simulink model "Select_PI_for_FOC_of_IM"  (R2017b)
settings: Solver=FixedStepDiscrete  StartTime=0.0  StopTime=10.0  FixedStep=Ts  MaxStep=1e-4  RelTol=1e-3
InitFcn:
  | Ts = 2e-5; Fsw = 2e3;
  | %Motor 1
  | %===========================
  | %Pn = 15e3; Nn = 1460; Tn = 9.55*Pn/Nn;
  | %Rs = 0.2147; Lls = 0.000991;
  | %Rr = 0.2205; Llr = 0.000991;
  | %Lm = 0.06419;
  | %Ls = Lls + Lm;
  | %Lr = Llr + Lm;
  | %P = 4;
  | %J = 0.102;  B = 0.009541;
  | %===========================
  | % Motor 2
  | %===========================
  | Pn = 7.5e3; Nn = 1440; Tn = 9.55*Pn/Nn;
  | Rs = 0.7384; Lls = 0.003045;
  | Rr = 0.7402; Llr = 0.003045;
  | Lm = 0.1241;
  | Ls = Lls + Lm;
  | Lr = Llr + Lm;
  | P = 4;  %poles
  | J = 0.0343;  B = 0.000503;
  | %===========================
  | Tor = (Llr+Lm) /Rr;
  | sigma = 1 - Lm*Lm/(Ls*Lr);
  | Kpdq = (Rs+Rr*(Lm/Lr)^2)*2*pi*50;
  | Kidq  = sigma*Ls*2*pi*50;
  | Ids_ref = 220*sqrt(2)/sqrt(Rs^2+(2*pi*50*Ls)^2);
  | KT = (3/2)*(P/2)*(Lm^2/Lr)*Ids_ref;
  | %Kpw = J*2*pi*50/KT;
  | %Kiw = Kpw*2*pi*50/5;
  | Zt = 0.8; W_n = 2*pi*5;
  | Kpw = (2*Zt*W_n*J-B);
  | Kiw  = (J*W_n^2);
  | Nze = 1e-3;
undefined symbols (not defined in the file): DiscIntNeverNeededParam, Vdc
libraries: powerlib x4, powerlib_meascontrol x3, peGeneralControl x1
settings Model: Creator=ADMIN  LastModifiedBy=ADMIN

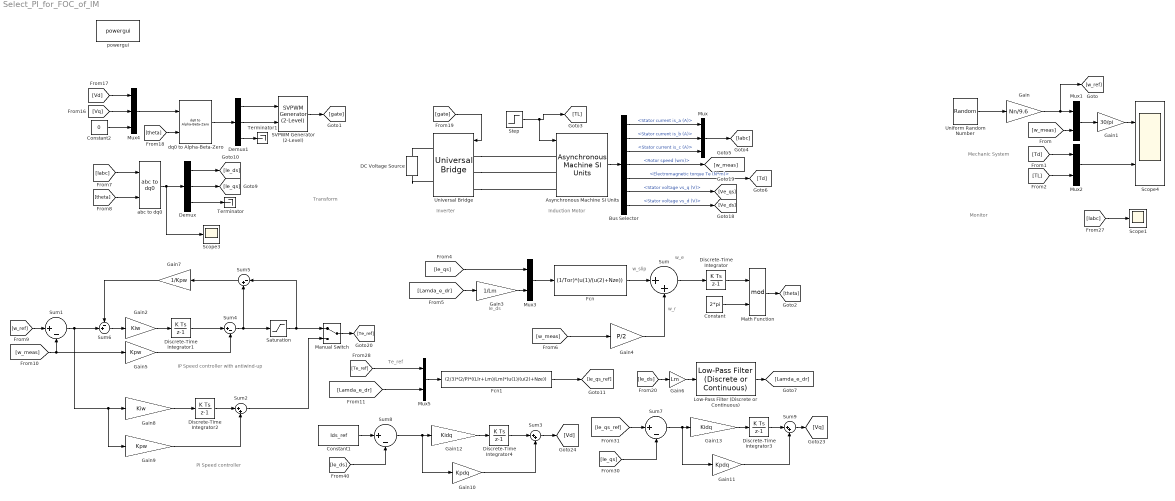
== system Select_PI_for_FOC_of_IM ==
  note: Monitor
  note: Induction Motor
  note: Transform
  note: Inverter
  note: Mechanic System
  note: Te_ref
  note: Ie_ds
  note: w_r
  note: w_slip
  note: w_e
  note: PI Speed controller
  note: IP Speed controller with antiwind-up
  Asynchronous Machine SI Units : powerlib/Machines/Asynchronous Machine SI Units  RotorType=Squirrel-cage  PresetModel="16:  10 HP (7.5KW)  400 V 50Hz 1440 RPM"  MechanicalLoad=Torque Tm  ShowDetailedParameters=on  ReferenceFrame=Synchronous  Units=SI  MeasurementBus=off  NominalParameters=[7500 400 50]  Stator=[0.7384 0.003045]  Rotor=[0.7402 0.003045]  Cage1=[0.4155 0.002066]  Cage2=[0.4168 0.0003495]  Lm=0.1241  Mechanical=[0.0343 0.000503 2]  PolePairs=2  InitialConditions=[1 0 0 0 0 0 0 0]  SimulateSaturation=off  Saturation=[14.03593122, 27.81365428, 53.79336849, 72.68890987, 97.98006896, 148.6815601, 215.7428561, 302.9841135, 428.7778367 ; 230, 322, 414, 460, 506, 552, 598, 644, 690]  LoadFlowParameters=1492000  TsPowergui=0  TsBlock=-1  IterativeModel=Trapezoidal non iterative  IterativeDiscreteModel=Trapezoidal non iterative  Pmec=0
  Bus Selector : BusSelector  OutputSignals=Stator measurements.Stator current is_a (A),Stator measurements.Stator current is_b (A),Stator measurements.Stator current is_c (A),Mechanical.Rotor speed (wm),Mechanical.Electromagnetic torque Te (N*m),Stator measurements.Stator voltage vs_q (V),Stator measurements.Stator voltage vs_d (V)
  Constant : Constant  Value=2*pi
  Constant1 : Constant  Value=Ids_ref
  Constant2 : Constant  Value=0
  DC Voltage Source : powerlib/Electrical Sources/DC Voltage Source  Amplitude=Vdc  Measurements=None
  Demux : Demux  Outputs=3
  Demux1 : Demux  Outputs=3
  Discrete-Time Integrator{,1..4} (5 alike) : DiscreteIntegrator  InitialConditionSetting=State (most efficient)  SampleTime=-1  ICPrevOutput=DiscIntNeverNeededParam  ICPrevScaledInput=DiscIntNeverNeededParam
  Fcn : Fcn  Expr=(1/Tor)*(u(1)/(u(2)+Nze))
  Fcn1 : Fcn  Expr=(2/3)*(2/P)*((Llr+Lm)/Lm)*(u(1)/(u(2)+Nze))
  Gain : Gain  Gain=Nn/9.6
  Gain1 : Gain  Gain=30/pi
  Gain10 : Gain  Gain=Kpdq
  Gain11 : Gain  Gain=Kpdq
  Gain12 : Gain  Gain=Kidq
  Gain13 : Gain  Gain=Kidq
  Gain2 : Gain  Gain=Kiw
  Gain3 : Gain  Gain=1/Lm
  Gain4 : Gain  Gain=P/2
  Gain5 : Gain  Gain=Kpw
  Gain6 : Gain  Gain=Lm
  Gain7 : Gain  Gain=1/Kpw
  Gain8 : Gain  Gain=Kiw
  Gain9 : Gain  Gain=Kpw
  Low-Pass Filter (Discrete or Continuous) : peGeneralControl/Low-Pass Filter (Discrete or Continuous)  K=1  T=Tor  B=inf  A=-inf  Ts=Ts
  Manual Switch : ManualSwitch
  Math Function : Math  Operator=mod  SaturateOnIntegerOverflow=on
  Mux : Mux  Inputs=3
  Mux{1..3,5} (4 alike) : Mux  Inputs=2
  Mux4 : Mux  Inputs=3
  SVPWM Generator (2-Level) : powerlib_meascontrol/Pulse & Signal Generators/SVPWM Generator (2-Level)  InputType=alpha-beta components  SwitchingPattern=Pattern #1  Fc=Fsw  ParUref=[0.8 -30 50]  Ts=Ts
      settings: SourceProductName=Simscape Power Systems  SourceProductBaseCode=PS
  Saturation : Saturate  UpperLimit=1.5*Tn  LowerLimit=-1.5*Tn
  Scope1 : Scope
  Scope3 : Scope
  Scope4 : Scope  NumInputPorts=2
  Step : Step  Time=5  Before=0.5*Tn  After=Tn  SampleTime=Ts
  Sum{,2..3,9} (4 alike) : Sum  Inputs=|++
  Sum{1,4,7..8} (4 alike) : Sum  Inputs=|+-
  Sum5 : Sum  Inputs=|-+
  Sum6 : Sum  Inputs=-+|
  Terminator : Terminator
  Terminator1 : Terminator
  Uniform Random Number : UniformRandomNumber  Minimum=0  Seed=5  SampleTime=2
  Universal Bridge : powerlib/Power Electronics/Universal Bridge  Arms=3  SnubberResistance=1e5  SnubberCapacitance=inf  Device=IGBT / Diodes  Ron=1e-3  Lon=0  ForwardVoltages="[  0  0  ]"  ForwardVoltage=0  GTOparameters=[ 10e-6 , 20e-6 ]  IGBTparameters=[ 1e-6 , 2e-6 ]  Measurements=None  Measurements_2=None  converterType=Rectifier
  abc to dq0 : powerlib_meascontrol/Transformations/abc to dq0  Alignment=90 degrees behind phase A axis
  dq0 to Alpha-Beta-Zero : powerlib_meascontrol/Transformations/dq0 to Alpha-Beta-Zero  Alignment=90 degrees behind phase A axis
      settings: SourceProductName=Simscape Power Systems  SourceProductBaseCode=PS
  powergui : powerlib/powergui  Priority=1  SimulationMode=Discrete  SampleTime=Ts  frequency=60  Iterations=50  frequencyindice=50  Pbase=100e6  ErrMax=1e-4  UnitsV=kV  UnitsW=MW  buscounter=0  FunctionMessages=off  echomessages=off  EnableUseOfTLC=off  CurrentSourceSwitches=off  DisableSnubberDevices=off  DisableRonSwitches=off  DisableVfSwitches=off  DisplayEquations=off  SolverType=Tustin/Backward Euler (TBE)  Interpol=off  ExternalGateDelay=off  methode=off  Ts=100  x0status=blocks  SPID=on  SwTol=0  HookPort=off  RestoreLinks=warning  ResistiveCurrentMeasurement=off  Frange=[0:2:500]  Ylog=off  Xlog=on  ShowGrid=off  save=off  variable=ZData  structure=IABC  ZoomFFT=off  StartTime=1.5  cycles=1  DisplayStyle=1  fundamental=6.7  FreqAxis=off  MaxFrequency=7000  frequencyindicesteady=1  RmsSteady=1  display=off
  wires:
  Step/1 -> [TL], Asynchronous Machine SI Units/1
  Demux/3 -> Terminator/1
  [TL] -> Mux2/2
  Fcn1/1 -> [Ie_qs_ref]
  Mux/1 -> [Iabc]
  Mux4/1 -> dq0 to Alpha-Beta-Zero/1
  dq0 to Alpha-Beta-Zero/1 -> Demux1/1
  Gain1/1 -> Scope4/1
  Demux1/1 -> SVPWM Generator (2-Level)/1
  [theta] -> abc to dq0/2
  Bus Selector/6 -> [Ve_qs]  "<Stator voltage vs_q (V)>"
  Saturation/1 -> Sum5/1, Manual Switch/1
  [gate] -> Universal Bridge/1
  Bus Selector/7 -> [Ve_ds]  "<Stator voltage vs_d (V)>"
  Demux/1 -> [Ie_ds]
  [w_meas] -> Gain4/1
  Demux1/2 -> SVPWM Generator (2-Level)/2
  Bus Selector/5 -> [Td]  "<Electromagnetic torque Te (N*m)>"
  Demux/2 -> [Ie_qs]
  Mux1/1 -> Gain1/1
  Low-Pass Filter (Discrete or Continuous)/1 -> [Lamda_e_dr]
  Asynchronous Machine SI Units/1 -> Bus Selector/1
  Bus Selector/4 -> [w_meas]  "<Rotor speed (wm)>"
  [Td] -> Mux2/1
  Mux2/1 -> Scope4/2
  [w_ref] -> Sum1/1
  Demux1/3 -> Terminator1/1
  Constant2/1 -> Mux4/3
  abc to dq0/1 -> Scope3/1, Demux/1
  [Vq] -> Mux4/2
  [Iabc] -> abc to dq0/1
  Bus Selector/1 -> Mux/1  "<Stator current is_a (A)>"
  [Iabc] -> Scope1/1
  Gain/1 -> [w_ref], Mux1/1
  [theta] -> dq0 to Alpha-Beta-Zero/2
  [w_meas] -> Mux1/2
  Bus Selector/2 -> Mux/2  "<Stator current is_b (A)>"
  SVPWM Generator (2-Level)/1 -> [gate]
  Uniform Random Number/1 -> Gain/1
  Bus Selector/3 -> Mux/3  "<Stator current is_c (A)>"
  Manual Switch/1 -> [Te_ref]
  [Vd] -> Mux4/1
  [Ie_ds] -> Gain6/1
  Gain6/1 -> Low-Pass Filter (Discrete or Continuous)/1
  [Lamda_e_dr] -> Mux5/2
  [Te_ref] -> Mux5/1
  Mux5/1 -> Fcn1/1
  [Lamda_e_dr] -> Gain3/1
  Math Function/1 -> [theta]
  Fcn/1 -> Sum/1
  [Ie_qs] -> Mux3/1
  Discrete-Time Integrator/1 -> Math Function/1
  Constant/1 -> Math Function/2
  Sum/1 -> Discrete-Time Integrator/1
  Mux3/1 -> Fcn/1
  Gain4/1 -> Sum/2
  Gain3/1 -> Mux3/2
  Gain5/1 -> Sum4/2
  Gain7/1 -> Sum6/1
  Sum5/1 -> Gain7/1
  Gain2/1 -> Discrete-Time Integrator1/1
  Sum6/1 -> Gain2/1
  Discrete-Time Integrator1/1 -> Sum4/1
  [w_meas] -> Gain5/1, Sum1/2
  Sum4/1 -> Sum5/2, Saturation/1
  Gain9/1 -> Sum2/2
  Sum1/1 -> Gain8/1, Gain9/1, Sum6/2
  Sum2/1 -> Manual Switch/2
  Gain8/1 -> Discrete-Time Integrator2/1
  Discrete-Time Integrator2/1 -> Sum2/1
  Sum9/1 -> [Vq]
  Gain10/1 -> Sum3/2
  [Ie_ds] -> Sum8/2
  Discrete-Time Integrator3/1 -> Sum9/1
  Constant1/1 -> Sum8/1
  [Ie_qs_ref] -> Sum7/1
  Gain11/1 -> Sum9/2
  Discrete-Time Integrator4/1 -> Sum3/1
  Sum8/1 -> Gain10/1, Gain12/1
  [Ie_qs] -> Sum7/2
  Gain12/1 -> Discrete-Time Integrator4/1
  Gain13/1 -> Discrete-Time Integrator3/1
  Sum3/1 -> [Vd]
  Sum7/1 -> Gain11/1, Gain13/1
  connections:
  Universal Bridge/LConn3 -- Asynchronous Machine SI Units/LConn3
  Universal Bridge/LConn2 -- Asynchronous Machine SI Units/LConn2
  DC Voltage Source/LConn1 -- Universal Bridge/RConn2
  Universal Bridge/LConn1 -- Asynchronous Machine SI Units/LConn1
  DC Voltage Source/RConn1 -- Universal Bridge/RConn1
